simulink model "trenl"  (Simulink 10.2)
settings: Solver=VariableStepAuto  StartTime=0.0  StopTime=10.0  RelTol=1e-3
undefined symbols (not defined in the file): Am, R, Ts
libraries: simulink x2, commanapbnd3 x2
settings Model: Creator=Robotcomp  LastModifiedBy=Robotcomp
settings DataIOCC: SaveFormat=Dataset  SignalLoggingSaveFormat=Dataset  ReturnWorkspaceOutputs=on
settings OptimizationCC: LifeSpan=auto
settings DebuggingCC: UnderspecifiedInitializationDetection=Simplified  MergeDetectMultiDrivingBlocksExec=error  FcnCallInpInsideContextMsg=error  SFUnexpectedBacktrackingDiag=error  SFNoUnconditionalDefaultTransitionDiag=error  SFExecutionAtInitializationDiag=warning  ArithmeticOperatorsInVariantConditions=error
settings HardwareCC: ProdBitPerPointer=64  ProdBitPerSizeT=64  ProdBitPerPtrDiffT=64  ProdLargestAtomicFloat=Float  ProdIntDivRoundTo=Zero  ProdEndianess=LittleEndian  ProdWordSize=64  ProdHWDeviceType=Intel->x86-64 (Windows64)
settings ModelReferenceCC: PropagateSignalLabelsOutOfModel=on
settings SFSimCC: SimUseLocalCustomCode=on  CustomCodeUndefinedFunction=FilterOut
settings RTWCC: RTWUseLocalCustomCode=on
settings CodeAppCC: StateflowObjectComments=off
settings GRTTargetCC: TargetLangStandard=C99 (ISO)  CombineOutputUpdateFcns=on  GRTInterface=off
settings ConfigComp: CovMetricSettings=dwe  CovSaveCumulativeToWorkspaceVar=off  CovSaveSingleToWorkspaceVar=off  CovExternalEMLEnable=on

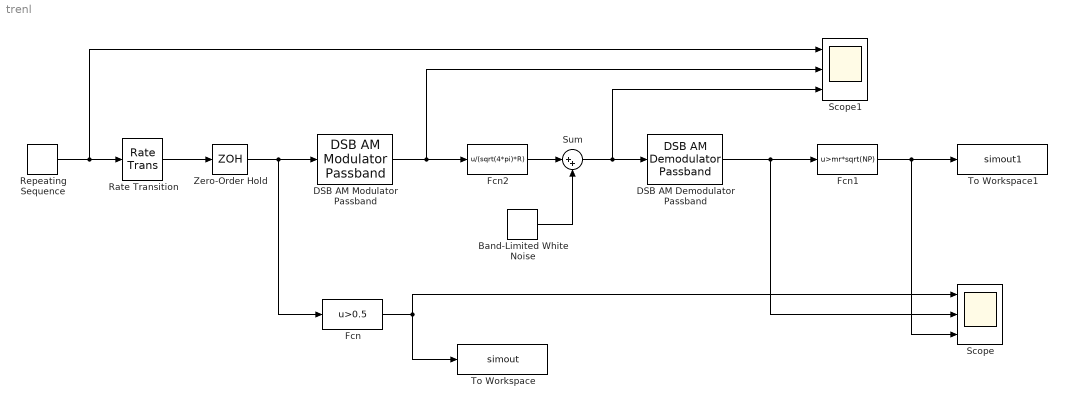
== system trenl ==
  Band-Limited White Noise : simulink/Sources/Band-Limited White Noise  Cov=NP  Ts=Ts  seed=to
  DSB AM Demodulator Passband : commanapbnd3/DSB AM Demodulator Passband  Fc=Hz  Ph=0  method=Butterworth  n=1  cf=100  Rp=0.1  Rs=50  Offset=1
      settings: SourceProductBaseCode=CM
  DSB AM Modulator Passband : commanapbnd3/DSB AM Modulator Passband  Fc=Hz  Ph=0  Offset=1
      settings: SourceProductBaseCode=CM
  Fcn : Fcn  Expr=u>0.5
  Fcn1 : Fcn  Expr=u>mr*sqrt(NP)
  Fcn2 : Fcn  Expr=u/(sqrt(4*pi)*R)
  Rate Transition : RateTransition  OutPortSampleTime=Ts
  Repeating Sequence : simulink/Sources/Repeating Sequence  rep_seq_t=[0 1]  rep_seq_y=[0 Am]
  Scope : Scope  NumInputPorts=3
  Scope1 : Scope  NumInputPorts=3
  Sum : Sum  Inputs=|++
  To Workspace : ToWorkspace  VariableName=simout  SampleTime=1
  To Workspace1 : ToWorkspace  VariableName=simout1  SampleTime=1
  Zero-Order Hold : ZeroOrderHold  SampleTime=Ts
  wires:
  Repeating Sequence/1 -> Scope1/1, Rate Transition/1
  Rate Transition/1 -> Zero-Order Hold/1
  Zero-Order Hold/1 -> DSB AM Modulator Passband/1, Fcn/1
  DSB AM Modulator Passband/1 -> Scope1/2, Fcn2/1
  Sum/1 -> Scope1/3, DSB AM Demodulator Passband/1
  Band-Limited White Noise/1 -> Sum/2
  DSB AM Demodulator Passband/1 -> Fcn1/1, Scope/2
  Fcn/1 -> Scope/1, To Workspace/1
  Fcn2/1 -> Sum/1
  Fcn1/1 -> To Workspace1/1, Scope/3
